simulink model "AnalogEE"  (Simulink 8.4)
settings: Solver=ode45  StartTime=0.0  StopTime=3  RelTol=1e-3
libraries: NeuroModelerLibrary x4
settings Model: Creator=user  LastModifiedBy=Tim

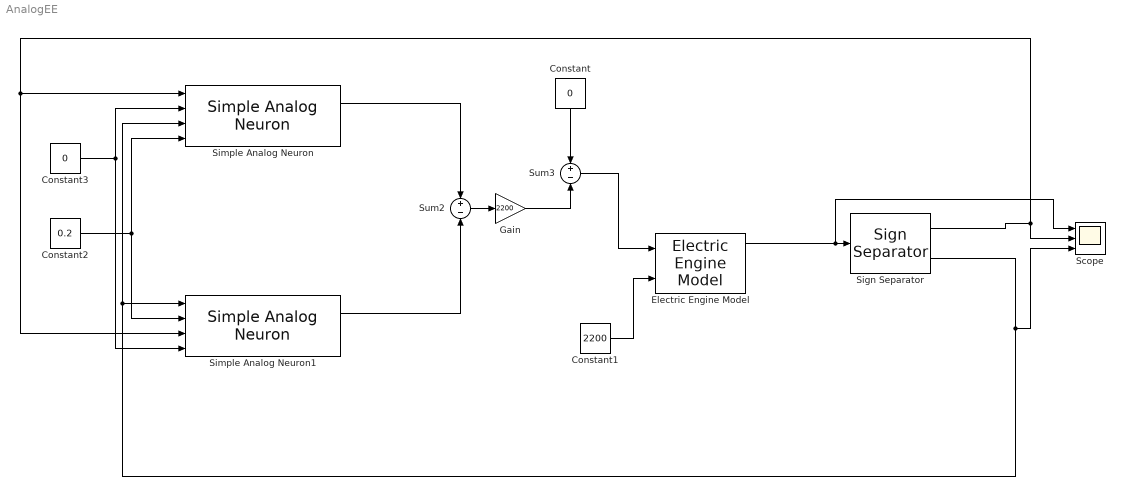
== system AnalogEE ==
  Constant : Constant  Value=0
  Constant1 : Constant  Value=2200
  Constant2 : Constant  Value=0.2
  Constant3 : Constant  Value=0
  Electric Engine Model : NeuroModelerLibrary/Support/Electric Engine Model
  Gain : Gain  Gain=2200  SaturateOnIntegerOverflow=on  OutDataTypeStr=Inherit: Same as input  ParamDataTypeStr=Inherit: Same as input
  Scope : Scope  NumInputPorts=3
      settings: TimeRange=3  YMin=-0.2~0~0  YMax=0.2~0.2~0.1
  Sign Separator : NeuroModelerLibrary/Support/Sign Separator
  Simple Analog Neuron : NeuroModelerLibrary/Analog Simple Cells/Simple Analog Neuron
  Simple Analog Neuron1 : NeuroModelerLibrary/Analog Simple Cells/Simple Analog Neuron
  Sum2 : Sum  Inputs=+-  SaturateOnIntegerOverflow=on  InputSameDT=on  OutDataTypeStr=Inherit: Same as first input
  Sum3 : Sum  Inputs=+-  SaturateOnIntegerOverflow=on  InputSameDT=on  OutDataTypeStr=Inherit: Same as first input
  wires:
  Sum3/1 -> Electric Engine Model/1
  Gain/1 -> Sum3/2
  Constant/1 -> Sum3/1
  Electric Engine Model/1 -> Sign Separator/1, Scope/1
  Constant1/1 -> Electric Engine Model/2
  Constant2/1 -> Simple Analog Neuron1/2, Simple Analog Neuron/4
  Constant3/1 -> Simple Analog Neuron1/4, Simple Analog Neuron/2
  Sum2/1 -> Gain/1
  Simple Analog Neuron/1 -> Sum2/1
  Simple Analog Neuron1/1 -> Sum2/2
  Sign Separator/1 -> Simple Analog Neuron1/3, Simple Analog Neuron/1, Scope/2
  Sign Separator/2 -> Scope/3, Simple Analog Neuron1/1, Simple Analog Neuron/3
